simulink model "demo_fft"  (R2023a)
settings: Solver=FixedStepDiscrete  StartTime=0.0  StopTime=dspb_fft.SimulationTime  FixedStep=1  RelTol=1e-3  EnableMultiTasking=on
PreLoadFcn:
  | warning off Simulink:Commands:SetParamLinkChangeWarn
  | warning off Simulink:Commands:LoadMdlParameterizedLink
  | warning off Simulink:SL_SetParamLinkChangeWarn
  | warning off Simulink:SL_LoadMdlParameterizedLink
  | setup_demo_fft;
InitFcn:
  | setup_demo_fft;
StopFcn:
  | analyze_subchannel_fft(...
  |      dspb_fft.FFTsize, ...
  |      dspb_fft.subchannels, ...
  |      dspb_fft.IFFT, ...
  |      dspb_fft.bit_reversed, ...
  |      dspb_fft.bit_reversed, ...
  |      v_in, chan_in,  x_in, ...
  |      v_out,chan_out, z_out);
undefined symbols (not defined in the file or in its folder): AdvDSPBChannelOutDisplay, dspb_fft, dspba_ChannelInVis, dspba_ChannelOutVis, dspba_internal_get_channel_ports, latency, value
libraries: DSPBAPrim x19, DSPBABase x4, DSPBAVectorUtil x3, simulink x3, DspbAdvFftLibrary x2
Description:
  | This design example implements a Fast Fourier Transform.
settings Model: Creator=lrigby  LastModifiedBy=5g
settings SolverCC: AlgebraicLoopSolver=TrustRegion
settings DataIOCC: LimitDataPoints=on  SaveFormat=Array  SignalLoggingSaveFormat=ModelDataLogs  ReturnWorkspaceOutputs=off
settings OptimizationCC: ExpressionDepthLimit=2147483647  InitFltsAndDblsToZero=on  LifeSpan=inf
settings DebuggingCC: SaveWithParameterizedLinksMsg=none  UnderspecifiedInitializationDetection=Classic  MergeDetectMultiDrivingBlocksExec=none  SignalResolutionControl=TryResolveAllWithWarning  SolverPrmCheckMsg=warning  ParameterPrecisionLossMsg=none  FcnCallInpInsideContextMsg=warning  UnconnectedInputMsg=warning  UnconnectedOutputMsg=warning  UnconnectedLineMsg=warning  StateNameClashWarn=warning  SFUnexpectedBacktrackingDiag=warning  SFNoUnconditionalDefaultTransitionDiag=warning  SFExecutionAtInitializationDiag=none  ArithmeticOperatorsInVariantConditions=warning
settings HardwareCC: ProdBitPerPointer=32  ProdBitPerSizeT=32  ProdBitPerPtrDiffT=32  ProdLargestAtomicFloat=None  ProdIntDivRoundTo=Undefined  ProdEndianess=Unspecified  ProdWordSize=32  ProdHWDeviceType=ASIC/FPGA  TargetBitPerLong=64  TargetBitPerPointer=64  TargetBitPerSizeT=64  TargetBitPerPtrDiffT=64  TargetLongLongMode=on  TargetIntDivRoundTo=Zero  TargetEndianess=LittleEndian  TargetWordSize=64  TargetHWDeviceType=MATLAB Host  ProdEqTarget=off
settings ModelReferenceCC: EnableRefExpFcnMdlSchedulingChecks=on  PropagateSignalLabelsOutOfModel=off
settings SFSimCC: SimUseLocalCustomCode=off  SimParseCustomCode=off  CustomCodeUndefinedFunction=UseInterfaceOnly
settings RTWCC: RTWUseLocalCustomCode=off  DLArmComputeVersion=19.05
settings CodeAppCC: StateflowObjectComments=on
settings GRTTargetCC: TargetFcnLib=ansi_tfl_tmw.mat  TargetLangStandard=C89/C90 (ANSI)  CombineOutputUpdateFcns=off  GRTInterface=on
settings ConfigComp: CovMetricSettings=dw  CovSaveCumulativeToWorkspaceVar=on  CovSaveSingleToWorkspaceVar=on  CovExternalEMLEnable=off

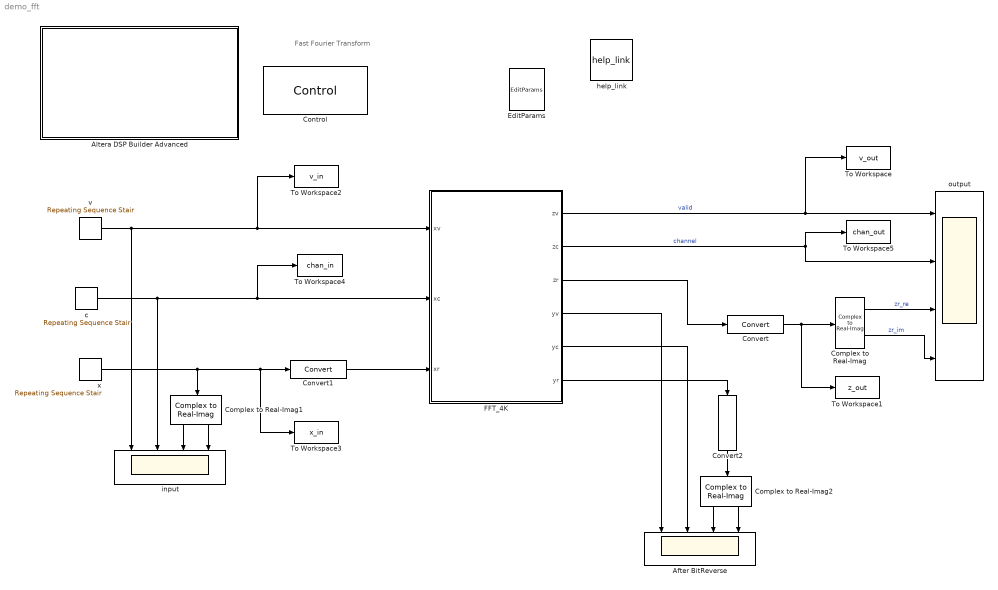
== system demo_fft ==
  note: Fast Fourier Transform
  After BitReverse : Scope  NumInputPorts=4
  Altera DSP Builder Advanced : Subsystem  mask(DSP Builder Advanced Blockset Ignored Block){}
      settings: OpenFcn=web('http://www.altera.com', '-new');
      mask Display: image(imread('intellogo.tif'));
  Complex to Real-Imag : DSPBAVectorUtil/Complex to Real-Imag
  Complex to Real-Imag1 : DSPBAVectorUtil/Complex to Real-Imag
  Complex to Real-Imag2 : DSPBAVectorUtil/Complex to Real-Imag
  Control : DSPBABase/Control  generate=on  language=VHDL  destination=rtl  make_full_path=off  path_is_relative=on  autotestbench=on  signaldepth=2  coveragetestbench=off  logs=off  spacewidth=2  spacenum=1  addrwidth=10  datawidth=16  dataendian=Big Endian  hierarchicalnames=on  ramThresholdBits=-1  distRamThresholdBits=-1  mlabThresholdBits=-1  hardMultiplierThresholdLuts=-1  version=20090407  errorOnChanMismatch=1  errorOnGPIOMismatch=0  importModelsimResults=0  cycleAccurate=off  reinterpretCastMult=off  paramFile=demo_fft_params.xml
  Convert : DSPBAPrim/Convert  primtype=convert  nInputs=1  nOutputs=1  omode=double  otype=sfix(16)  scale=2^-15  rndmethod=Unbiased  factor=1  satmethod=None  shift_vec=[0 1 2 -1]  value=round([0:255]/17)  inPortNames=[' '; ' ';]  outPortNames=[' '; 'c']  dspbaimage=dspba_prim_wide.svg  text=fprintf('convert');  style=Optimised  visibilities=8+64+256+2^17  clipdetect=off  floatPrecision=float32_m23  advOptions=[]  version=20211007
  Convert1 : DSPBAPrim/Convert  primtype=convert  nInputs=1  nOutputs=1  omode=Specify via dialog  otype=sfix(16)  scale=2^-14  rndmethod=Unbiased  factor=1  satmethod=None  shift_vec=[0 1 2 -1]  value=round([0:255]/17)  inPortNames=[' '; ' ';]  outPortNames=[' '; 'c']  dspbaimage=dspba_prim_wide.svg  text=fprintf('convert');  style=Optimised  visibilities=8+64+256+2^17  clipdetect=off  floatPrecision=float32_m23  advOptions=[]  version=20211007
  Convert2 : DSPBAPrim/Convert  primtype=convert  nInputs=1  nOutputs=1  omode=double  otype=sfix(16)  scale=2^-15  rndmethod=Unbiased  factor=1  satmethod=None  shift_vec=[0 1 2 -1]  value=round([0:255]/17)  inPortNames=[' '; ' ';]  outPortNames=[' '; 'c']  dspbaimage=dspba_prim_wide.svg  text=fprintf('convert');  style=Optimised  visibilities=8+64+256+2^17  clipdetect=off  floatPrecision=float32_m23  advOptions=[]  version=20211007
  EditParams : DSPBABase/EditParams  version=20090407
  FFT_4K : Subsystem
  To Workspace : ToWorkspace  VariableName=v_out  SampleTime=-1
  To Workspace1 : ToWorkspace  VariableName=z_out  SampleTime=-1
  To Workspace2 : ToWorkspace  VariableName=v_in  SampleTime=-1
  To Workspace3 : ToWorkspace  VariableName=x_in  SampleTime=-1
  To Workspace4 : ToWorkspace  VariableName=chan_in  SampleTime=-1
  To Workspace5 : ToWorkspace  VariableName=chan_out  SampleTime=-1
  c : simulink/Sources/Repeating Sequence Stair  OutValues=dspb_fft.channel_in  tsamp=dspb_fft.SampleTime  OutMin=[]  OutMax=[]  OutDataTypeStr=fixdt(0,8,0)  OutputDataTypeScalingMode=Specify via dialog  OutDataType=uint(8)  ConRadixGroup=Use specified scaling  OutScaling=2^-15
  help_link : DSPBABase/help_link  version=20090407
  input : Scope  NumInputPorts=4
  output : Scope  NumInputPorts=4
  v : simulink/Sources/Repeating Sequence Stair  OutValues=dspb_fft.valid_in  tsamp=dspb_fft.SampleTime  OutMin=[]  OutMax=[]  OutDataTypeStr=fixdt('boolean')  OutputDataTypeScalingMode=Specify via dialog  OutDataType=fixdt('boolean')  ConRadixGroup=Best Precision: Vector-wise  OutScaling=[]
  x : simulink/Sources/Repeating Sequence Stair  OutValues=dspb_fft.x_in  tsamp=dspb_fft.SampleTime  OutMin=[]  OutMax=[]  OutDataTypeStr=double  OutputDataTypeScalingMode=double  OutDataType=dspb_fft.InputType  ConRadixGroup=Best Precision: Vector-wise  OutScaling=[]
  wires:
  v/1 -> input/1, FFT_4K/1(xv), To Workspace2/1
  c/1 -> input/2, To Workspace4/1, FFT_4K/2(xc)
  x/1 -> To Workspace3/1, Convert1/1, Complex to Real-Imag1/1
  FFT_4K/3(zr) -> Convert/1
  Complex to Real-Imag/1 -> output/3  "zr_re"
  Complex to Real-Imag/2 -> output/4  "zr_im"
  Complex to Real-Imag1/1 -> input/3
  Complex to Real-Imag1/2 -> input/4
  Convert/1 -> Complex to Real-Imag/1, To Workspace1/1
  Convert1/1 -> FFT_4K/3(xr)
  FFT_4K/4(yv) -> After BitReverse/1
  FFT_4K/5(yc) -> After BitReverse/2
  FFT_4K/6(yr) -> Convert2/1
  Complex to Real-Imag2/1 -> After BitReverse/3
  Complex to Real-Imag2/2 -> After BitReverse/4
  Convert2/1 -> Complex to Real-Imag2/1
  FFT_4K/1(zv) -> output/1, To Workspace/1  "valid"
  FFT_4K/2(zc) -> output/2, To Workspace5/1  "channel"

== system demo_fft/Altera DSP Builder Advanced ==

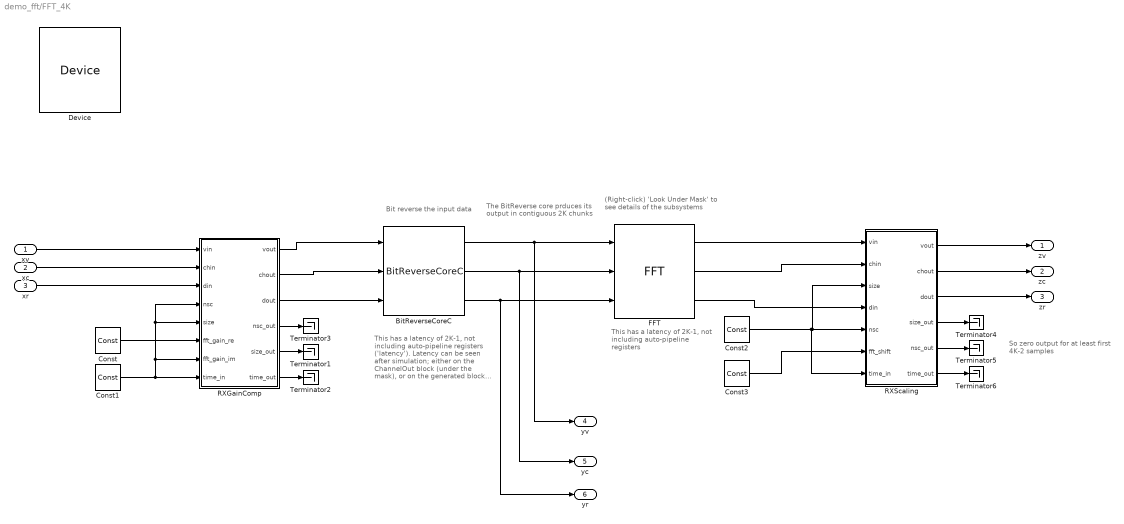
== system demo_fft/FFT_4K ==
  note: Bit reverse the input data
  note: This has a latency of 2K-1,
      | not including auto-pipeline
      | registers ('latency'). Latency
      | can be seen after simulation;
      | either on the ChannelOut block
      | (under the mask), or on the
      | generated block help.
  note: This has a latency of 2K-1,
      | not including auto-pipeline
      | registers
  note: So zero output for at
      | least first 4K-2 samples
  note: (Right-click) 'Look Under Mask'
      | to see details of the subsystems
  note: The BitReverse core prduces its
      | output in contiguous 2K chunks
  xv : Inport
  xc : Inport  Port=2
  xr : Inport  Port=3
  BitReverseCoreC : DspbAdvFftLibrary/Radix2/BitReverseCoreC  N=dspb_fft.FFTsize  subchannels=dspb_fft.subchannels
      link override ChannelOut: value=1  latency=6  nInputs=dspba_internal_get_channel_ports(gcb, 'inputs')  nOutputs=dspba_internal_get_channel_ports(gcb, 'outputs')  packetBeginEnabled=off  version=20140818
  Const : DSPBAPrim/Const  primtype=const  nInputs=0  nOutputs=1  omode=Specify via dialog  otype=sfix(16)  scale=2^-13  rndmethod=Unbiased  factor=1  satmethod=Symmetric  shift_vec=[0 1 2 -1]  value=1  inPortNames=['+'; '+';]  outPortNames=[' ']  dspbaimage=dspba_prim.svg  text=fprintf('%s', num2str(value));  style=Optimised  visibilities=8 + 1024  floatPrecision=float32_m23  warnSaturation=on  version=20211007  SampleTime=inf
  Const1 : DSPBAPrim/Const  primtype=const  nInputs=0  nOutputs=1  omode=Specify via dialog  otype=sfix(16)  scale=2^-13  rndmethod=Unbiased  factor=1  satmethod=Symmetric  shift_vec=[0 1 2 -1]  value=0  inPortNames=['+'; '+';]  outPortNames=[' ']  dspbaimage=dspba_prim.svg  text=fprintf('%s', num2str(value));  style=Optimised  visibilities=8 + 1024  floatPrecision=float32_m23  warnSaturation=on  version=20211007  SampleTime=inf
  Const2 : DSPBAPrim/Const  primtype=const  nInputs=0  nOutputs=1  omode=Specify via dialog  otype=sfix(16)  scale=2^-13  rndmethod=Unbiased  factor=1  satmethod=Symmetric  shift_vec=[0 1 2 -1]  value=0  inPortNames=['+'; '+';]  outPortNames=[' ']  dspbaimage=dspba_prim.svg  text=fprintf('%s', num2str(value));  style=Optimised  visibilities=8 + 1024  floatPrecision=float32_m23  warnSaturation=on  version=20211007  SampleTime=inf
  Const3 : DSPBAPrim/Const  primtype=const  nInputs=0  nOutputs=1  omode=Specify via dialog  otype=ufix(4)  scale=1  rndmethod=Unbiased  factor=1  satmethod=Symmetric  shift_vec=[0 1 2 -1]  value=0  inPortNames=['+'; '+';]  outPortNames=[' ']  dspbaimage=dspba_prim.svg  text=fprintf('%s', num2str(value));  style=Optimised  visibilities=8 + 1024  floatPrecision=float32_m23  warnSaturation=on  version=20211007  SampleTime=inf
  Device : DSPBABase/Device  family=Arria 10  stratix4device=Stratix IV E  hardcopy4device=HardCopy IV E  stratix5device=Stratix V GX  device=AUTO  speed=-3  stratixSpeed=-5  stratix2Speed=-3  stratix3Speed=-3  stratix4gxSpeed=-2  stratix4gtSpeed=-1  cyclone2Speed=-6  cyclone3Speed=-6  arria2Speed=-4  cyclone4eSpeed=-8  stratix5Speed=-3  arria5Speed=-4  arriaSpeed=-6  cyclone3lsSpeed=-7  cyclone5Speed=-6  arria2gzSpeed=-3  nightFurySpeed=-2  ecp2Speed=-7  hardcopycompat=off  version=20140217  max10flashmode=off  max10nomeminit=off
  FFT : DspbAdvFftLibrary/Common/FFT  IFFT=dspb_fft.IFFT  subchannels=dspb_fft.subchannels  br_in=~dspb_fft.bit_reversed  N=dspb_fft.N  in_type=dspb_fft.input_type  type_strings=dspb_fft.type_strings  faithful=true
      link override ChannelOut1: nInputs=dspba_internal_get_channel_ports(gcb, 'inputs')  nOutputs=dspba_internal_get_channel_ports(gcb, 'outputs')  value=1  packetBeginEnabled=off  latency=35  version=20140818
  RXGainComp : Subsystem  AncestorBlock=lib_lowphy/FFT_S2B/SignalProcessing/RXGainComp
  RXScaling : Subsystem
  Terminator{1..6} (6 alike) : Terminator
  zv : Outport
  zc : Outport  Port=2
  zr : Outport  Port=3
  yv : Outport  Port=4
  yc : Outport  Port=5
  yr : Outport  Port=6
  wires:
  BitReverseCoreC/1 -> yv/1, FFT/1
  BitReverseCoreC/2 -> FFT/2, yc/1
  BitReverseCoreC/3 -> FFT/3, yr/1
  Const/1 -> RXGainComp/6(fft_gain_re)
  Const1/1 -> RXGainComp/8(time_in), RXGainComp/4(nsc), RXGainComp/5(size), RXGainComp/7(fft_gain_im)
  RXGainComp/6(time_out) -> Terminator2/1
  RXGainComp/5(size_out) -> Terminator1/1
  RXGainComp/4(nsc_out) -> Terminator3/1
  Const2/1 -> RXScaling/7(time_in), RXScaling/3(size), RXScaling/5(nsc)
  RXScaling/4(size_out) -> Terminator4/1
  RXScaling/5(nsc_out) -> Terminator5/1
  RXScaling/6(time_out) -> Terminator6/1
  xv/1 -> RXGainComp/1(vin)
  xc/1 -> RXGainComp/2(chin)
  RXGainComp/1(vout) -> BitReverseCoreC/1
  RXGainComp/2(chout) -> BitReverseCoreC/2
  RXGainComp/3(dout) -> BitReverseCoreC/3
  Const3/1 -> RXScaling/6(fft_shift)
  xr/1 -> RXGainComp/3(din)
  FFT/1 -> RXScaling/1(vin)
  FFT/2 -> RXScaling/2(chin)
  FFT/3 -> RXScaling/4(din)
  RXScaling/1(vout) -> zv/1
  RXScaling/2(chout) -> zc/1
  RXScaling/3(dout) -> zr/1

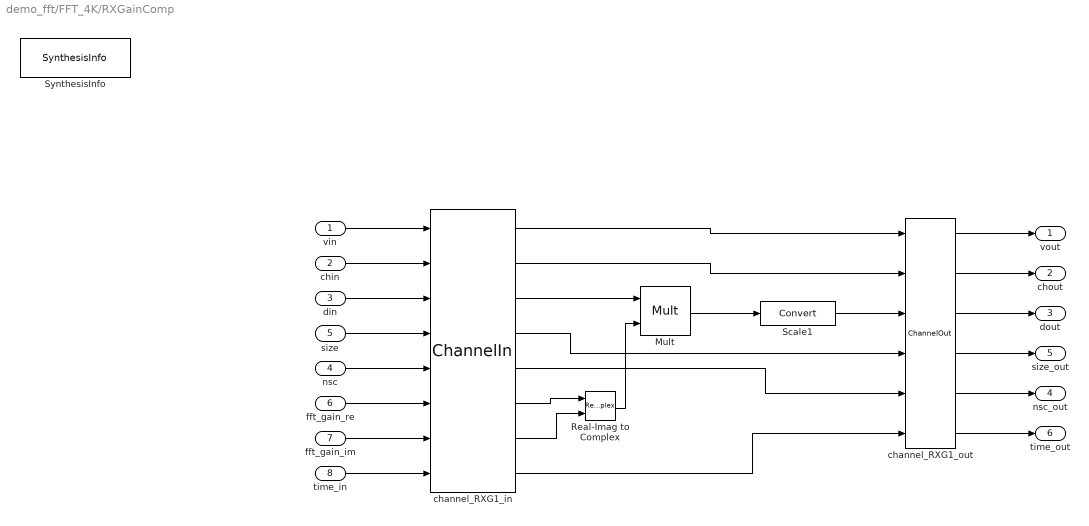
== system demo_fft/FFT_4K/RXGainComp ==
  vin : Inport
  chin : Inport  Port=2
  din : Inport  Port=3
  nsc : Inport  Port=4
  size : Inport  Port=5
  fft_gain_re : Inport  Port=6
  fft_gain_im : Inport  Port=7
  time_in : Inport  Port=8
  Mult : DSPBAPrim/Mult  primtype=mult  nInputs=2  nOutputs=1  omode=Inherit via internal rule  otype=sfix(16)  scale=2^-15  rndmethod=Unbiased  factor=1  satmethod=Symmetric  shift_vec=[0 1 2 -1]  value=0  inPortNames=[' '; ' ';]  outPortNames=[' ']  dspbaimage=dspba_prim.svg  text=fprintf('X');  style=Optimised  visibilities=8+2^18+2^19  floatPrecision=float32_m23  floatRounding=correct  advOptions=[]  version=20211007
  Real-Imag to Complex : RealImagToComplex
  Scale1 : DSPBAPrim/Convert  primtype=convert  nInputs=1  nOutputs=1  omode=Specify via dialog  otype=sfix(16)  scale=2^-14  rndmethod=Biased  factor=1  satmethod=Symmetric  shift_vec=[0 1 2 -1]  value=round([0:255]/17)  inPortNames=[' '; ' ';]  outPortNames=[' '; 'c']  dspbaimage=dspba_prim_wide.svg  text=fprintf('convert');  style=Optimised  visibilities=8+64+256+2^17  clipdetect=off  floatPrecision=float32_m23  advOptions=[]  version=20211007
  SynthesisInfo : DSPBAPrim/SynthesisInfo  primtype=synthinfo  nInputs=0  nOutputs=0  omode=Inherit via internal rule  otype=sfix(16)  scale=2^-15  rndmethod=Truncate  factor=1  satmethod=Symmetric  shift_vec=[0 1 2 -1]  value=99  inPortNames=[' '; ' ';]  outPortNames=[' ']  dspbaimage=dspba_prim_ctrl.jpg  text=fprintf('Style=%s', style);  style=Scheduled  visibilities=2^17+2^18+2^19+2^20  constraintPair=None  constraintRelation=>  constraintLimit=2  modelRefSign=+  modelRef=''  showSchedule=off  simulationMode=Use Global Value  resetMinimization=Conditional - On for ChannelIn/Out only  version=20220106
  channel_RXG1_in : DSPBAPrim/ChannelIn  primtype=channelin  nInputs=dspba_internal_get_channel_ports(gcb)  nOutputs=dspba_internal_get_channel_ports(gcb)  omode=Inherit via internal rule  otype=sfix(16)  scale=2^-15  rndmethod=Unbiased  factor=1  satmethod=Symmetric  shift_vec=[0 1 2 -1]  value=6  inPortNames=['v'; 'c'; '0'; '1'; '2'; '3'; '4'; '5'; '6'; '7'; '8'; '9'; 'A'; 'B'; 'D'; 'E'; 'F'; 'G'; 'H'; 'I'; 'J'; 'K'; 'L'; 'M'; 'N'; 'O'; 'P'; 'Q'; 'R'; 'S'; 'T'; 'U'; 'W'; 'X'; 'Y'; 'Z']  outPortNames=['v'; 'c'; '0'; '1'; '2'; '3'; '4'; '5'; '6'; '7'; '8'; '9'; 'A'; 'B'; 'D'; 'E'; 'F'; 'G'; 'H'; 'I'; 'J'; 'K'; 'L'; 'M'; 'N'; 'O'; 'P'; 'Q'; 'R'; 'S'; 'T'; 'U'; 'W'; 'X'; 'Y'; 'Z']  dspbaimage=dspba_prim_channel_tall.svg  text=fprintf('In');  style=Optimised  dataSignals=6  foldingEnabled=off  channels=1  sampleRate=200  packetBeginPresent=off  packetBeginEnabled=off  visibilities=dspba_ChannelInVis(gcb)  scheduleOrigin=off  version=20211214
  channel_RXG1_out : DSPBAPrim/ChannelOut  primtype=channelout  nInputs=dspba_internal_get_channel_ports(gcb)  nOutputs=dspba_internal_get_channel_ports(gcb)  omode=Inherit via internal rule  otype=sfix(16)  scale=2^-15  rndmethod=Unbiased  factor=1  satmethod=Symmetric  shift_vec=[0 1 2 -1]  value=4  inPortNames=['v'; 'c'; '0'; '1'; '2'; '3'; '4'; '5'; '6'; '7'; '8'; '9'; 'A'; 'B'; 'D'; 'E'; 'F'; 'G'; 'H'; 'I'; 'J'; 'K'; 'L'; 'M'; 'N'; 'O'; 'P'; 'Q'; 'R'; 'S'; 'T'; 'U'; 'W'; 'X'; 'Y'; 'Z']  outPortNames=['v'; 'c'; '0'; '1'; '2'; '3'; '4'; '5'; '6'; '7'; '8'; '9'; 'A'; 'B'; 'D'; 'E'; 'F'; 'G'; 'H'; 'I'; 'J'; 'K'; 'L'; 'M'; 'N'; 'O'; 'P'; 'Q'; 'R'; 'S'; 'T'; 'U'; 'W'; 'X'; 'Y'; 'Z']  dspbaimage=dspba_prim_channel_tall.svg  text=fprintf('Out%s', AdvDSPBChannelOutDisplay(latency));  style=Optimised  dataSignals=4  foldingEnabled=off  channels=1  sampleRate=200  packetBeginPresent=off  packetBeginEnabled=off  visibilities=dspba_ChannelOutVis(gcb)  latency=5  version=20211214
  vout : Outport
  chout : Outport  Port=2
  dout : Outport  Port=3
  nsc_out : Outport  Port=4
  size_out : Outport  Port=5
  time_out : Outport  Port=6
  wires:
  Real-Imag to Complex/1 -> Mult/2
  channel_RXG1_in/6 -> Real-Imag to Complex/1
  channel_RXG1_out/6 -> time_out/1
  channel_RXG1_in/8 -> channel_RXG1_out/6
  time_in/1 -> channel_RXG1_in/8
  channel_RXG1_in/7 -> Real-Imag to Complex/2
  fft_gain_im/1 -> channel_RXG1_in/7
  fft_gain_re/1 -> channel_RXG1_in/6
  nsc/1 -> channel_RXG1_in/5
  size/1 -> channel_RXG1_in/4
  channel_RXG1_in/5 -> channel_RXG1_out/5
  channel_RXG1_in/4 -> channel_RXG1_out/4
  channel_RXG1_out/5 -> nsc_out/1
  channel_RXG1_out/4 -> size_out/1
  din/1 -> channel_RXG1_in/3
  vin/1 -> channel_RXG1_in/1
  chin/1 -> channel_RXG1_in/2
  channel_RXG1_in/3 -> Mult/1
  channel_RXG1_out/3 -> dout/1
  channel_RXG1_in/2 -> channel_RXG1_out/2
  channel_RXG1_in/1 -> channel_RXG1_out/1
  channel_RXG1_out/2 -> chout/1
  channel_RXG1_out/1 -> vout/1
  Mult/1 -> Scale1/1
  Scale1/1 -> channel_RXG1_out/3

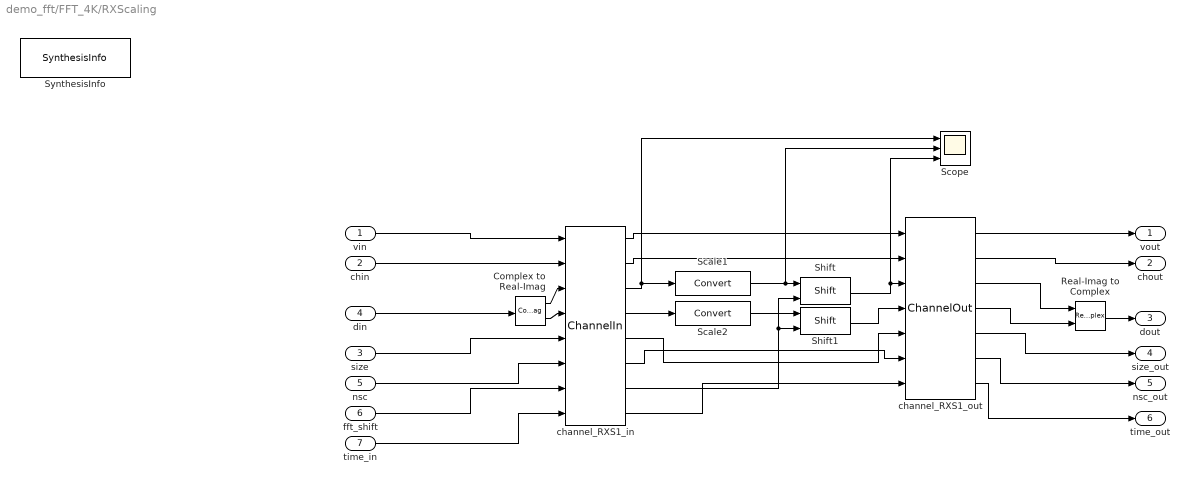
== system demo_fft/FFT_4K/RXScaling ==
  vin : Inport
  chin : Inport  Port=2
  size : Inport  Port=3
  din : Inport  Port=4
  nsc : Inport  Port=5
  fft_shift : Inport  Port=6
  time_in : Inport  Port=7
  Complex to Real-Imag : ComplexToRealImag
  Real-Imag to Complex : RealImagToComplex
  Scale1 : DSPBAPrim/Convert  primtype=convert  nInputs=1  nOutputs=1  omode=Specify via dialog  otype=sfix(16)  scale=2^-12  rndmethod=Biased  factor=1  satmethod=Symmetric  shift_vec=[0 1 2 -1]  value=round([0:255]/17)  inPortNames=[' '; ' ';]  outPortNames=[' '; 'c']  dspbaimage=dspba_prim_wide.svg  text=fprintf('convert');  style=Optimised  visibilities=8+64+256+2^17  clipdetect=off  floatPrecision=float32_m23  advOptions=[]  version=20211007
  Scale2 : DSPBAPrim/Convert  primtype=convert  nInputs=1  nOutputs=1  omode=Specify via dialog  otype=sfix(16)  scale=2^-12  rndmethod=Biased  factor=1  satmethod=Symmetric  shift_vec=[0 1 2 -1]  value=round([0:255]/17)  inPortNames=[' '; ' ';]  outPortNames=[' '; 'c']  dspbaimage=dspba_prim_wide.svg  text=fprintf('convert');  style=Optimised  visibilities=8+64+256+2^17  clipdetect=off  floatPrecision=float32_m23  advOptions=[]  version=20211007
  Scope : Scope  NumInputPorts=3
  Shift : DSPBAPrim/Shift  primtype=shift  nInputs=2  nOutputs=1  omode=Specify via dialog  otype=sfix(16)  scale=2^-12  rndmethod=Unbiased  factor=1  satmethod=Symmetric  shift_vec=[0 1 2 -1]  value=0  inPortNames=['a'; 'b';]  outPortNames=[' ']  dspbaimage=dspba_prim.svg  text=fprintf('a >> b');  style=Optimised  visibilities=8  version=20211007
  Shift1 : DSPBAPrim/Shift  primtype=shift  nInputs=2  nOutputs=1  omode=Specify via dialog  otype=sfix(16)  scale=2^-12  rndmethod=Unbiased  factor=1  satmethod=Symmetric  shift_vec=[0 1 2 -1]  value=0  inPortNames=['a'; 'b';]  outPortNames=[' ']  dspbaimage=dspba_prim.svg  text=fprintf('a >> b');  style=Optimised  visibilities=8  version=20211007
  SynthesisInfo : DSPBAPrim/SynthesisInfo  primtype=synthinfo  nInputs=0  nOutputs=0  omode=Inherit via internal rule  otype=sfix(16)  scale=2^-15  rndmethod=Truncate  factor=1  satmethod=Symmetric  shift_vec=[0 1 2 -1]  value=99  inPortNames=[' '; ' ';]  outPortNames=[' ']  dspbaimage=dspba_prim_ctrl.jpg  text=fprintf('Style=%s', style);  style=Scheduled  visibilities=2^17+2^18+2^19+2^20  constraintPair=None  constraintRelation=>  constraintLimit=2  modelRefSign=+  modelRef=''  showSchedule=off  simulationMode=Use Global Value  resetMinimization=Conditional - On for ChannelIn/Out only  version=20220106
  channel_RXS1_in : DSPBAPrim/ChannelIn  primtype=channelin  nInputs=dspba_internal_get_channel_ports(gcb)  nOutputs=dspba_internal_get_channel_ports(gcb)  omode=Inherit via internal rule  otype=sfix(16)  scale=2^-15  rndmethod=Unbiased  factor=1  satmethod=Symmetric  shift_vec=[0 1 2 -1]  value=6  inPortNames=['v'; 'c'; '0'; '1'; '2'; '3'; '4'; '5'; '6'; '7'; '8'; '9'; 'A'; 'B'; 'D'; 'E'; 'F'; 'G'; 'H'; 'I'; 'J'; 'K'; 'L'; 'M'; 'N'; 'O'; 'P'; 'Q'; 'R'; 'S'; 'T'; 'U'; 'W'; 'X'; 'Y'; 'Z']  outPortNames=['v'; 'c'; '0'; '1'; '2'; '3'; '4'; '5'; '6'; '7'; '8'; '9'; 'A'; 'B'; 'D'; 'E'; 'F'; 'G'; 'H'; 'I'; 'J'; 'K'; 'L'; 'M'; 'N'; 'O'; 'P'; 'Q'; 'R'; 'S'; 'T'; 'U'; 'W'; 'X'; 'Y'; 'Z']  dspbaimage=dspba_prim_channel_tall.svg  text=fprintf('In');  style=Optimised  dataSignals=6  foldingEnabled=off  channels=1  sampleRate=200  packetBeginPresent=off  packetBeginEnabled=off  visibilities=dspba_ChannelInVis(gcb)  scheduleOrigin=off  version=20211214
  channel_RXS1_out : DSPBAPrim/ChannelOut  primtype=channelout  nInputs=dspba_internal_get_channel_ports(gcb)  nOutputs=dspba_internal_get_channel_ports(gcb)  omode=Inherit via internal rule  otype=sfix(16)  scale=2^-15  rndmethod=Unbiased  factor=1  satmethod=Symmetric  shift_vec=[0 1 2 -1]  value=5  inPortNames=['v'; 'c'; '0'; '1'; '2'; '3'; '4'; '5'; '6'; '7'; '8'; '9'; 'A'; 'B'; 'D'; 'E'; 'F'; 'G'; 'H'; 'I'; 'J'; 'K'; 'L'; 'M'; 'N'; 'O'; 'P'; 'Q'; 'R'; 'S'; 'T'; 'U'; 'W'; 'X'; 'Y'; 'Z']  outPortNames=['v'; 'c'; '0'; '1'; '2'; '3'; '4'; '5'; '6'; '7'; '8'; '9'; 'A'; 'B'; 'D'; 'E'; 'F'; 'G'; 'H'; 'I'; 'J'; 'K'; 'L'; 'M'; 'N'; 'O'; 'P'; 'Q'; 'R'; 'S'; 'T'; 'U'; 'W'; 'X'; 'Y'; 'Z']  dspbaimage=dspba_prim_channel_tall.svg  text=fprintf('Out%s', AdvDSPBChannelOutDisplay(latency));  style=Optimised  dataSignals=5  foldingEnabled=off  channels=1  sampleRate=200  packetBeginPresent=off  packetBeginEnabled=off  visibilities=dspba_ChannelOutVis(gcb)  latency=2  version=20211214
  vout : Outport
  chout : Outport  Port=2
  dout : Outport  Port=3
  size_out : Outport  Port=4
  nsc_out : Outport  Port=5
  time_out : Outport  Port=6
  wires:
  channel_RXS1_out/7 -> time_out/1
  channel_RXS1_in/8 -> channel_RXS1_out/7
  time_in/1 -> channel_RXS1_in/8
  Scale2/1 -> Shift1/1
  Scale1/1 -> Shift/1, Scope/2
  channel_RXS1_in/7 -> Shift/2, Shift1/2
  channel_RXS1_in/4 -> Scale2/1
  channel_RXS1_in/3 -> Scale1/1, Scope/1
  fft_shift/1 -> channel_RXS1_in/7
  channel_RXS1_out/6 -> nsc_out/1
  channel_RXS1_in/6 -> channel_RXS1_out/6
  channel_RXS1_out/4 -> Real-Imag to Complex/2
  channel_RXS1_out/3 -> Real-Imag to Complex/1
  Real-Imag to Complex/1 -> dout/1
  din/1 -> Complex to Real-Imag/1
  Complex to Real-Imag/2 -> channel_RXS1_in/4
  Complex to Real-Imag/1 -> channel_RXS1_in/3
  nsc/1 -> channel_RXS1_in/6
  channel_RXS1_out/5 -> size_out/1
  channel_RXS1_in/5 -> channel_RXS1_out/5
  size/1 -> channel_RXS1_in/5
  Shift1/1 -> channel_RXS1_out/4
  Shift/1 -> channel_RXS1_out/3, Scope/3
  channel_RXS1_out/1 -> vout/1
  channel_RXS1_out/2 -> chout/1
  channel_RXS1_in/1 -> channel_RXS1_out/1
  channel_RXS1_in/2 -> channel_RXS1_out/2
  chin/1 -> channel_RXS1_in/2
  vin/1 -> channel_RXS1_in/1
